simulink model "singlestageSimu"  (R2015b)
settings: Solver=ode45  StartTime=0.0  StopTime=10.0  RelTol=1e-3
values from neighbouring files (symbols this model uses):
  b1n = 0.9    [directComputeTF.m]
  b2n = 0.8    [directComputeTF.m]
libraries: fl_lib x9, nesl_utility x3
settings Model: Creator=Jinwen  LastModifiedBy=Jinwen
settings DataIOCC: SaveFormat=Array
settings HardwareCC: ProdBitPerPointer=32  ProdLargestAtomicFloat=None  ProdIntDivRoundTo=Undefined  ProdEndianess=Unspecified  ProdWordSize=32  ProdHWDeviceType=32-bit Generic
settings GRTTargetCC: GeneratePreprocessorConditionals=Disable all
settings ConfigComp: CovModelRefEnable=Off

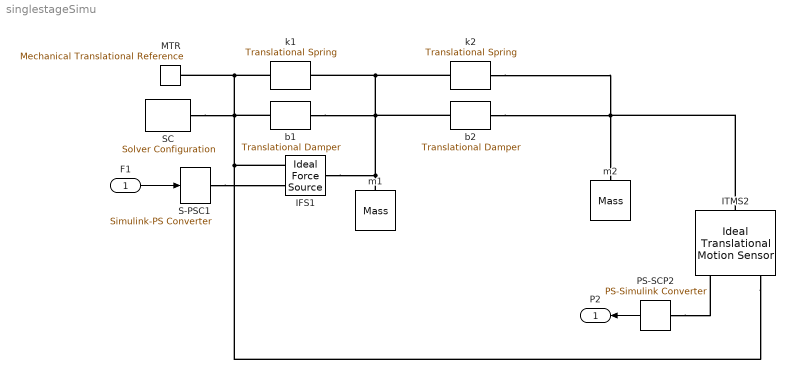
== system singlestageSimu ==
  F1 : Inport
  IFS1 : fl_lib/Mechanical/Mechanical Sources/Ideal Force Source
  ITMS2 : fl_lib/Mechanical/Mechanical Sensors/Ideal Translational Motion Sensor  offset=0 m
  MTR : fl_lib/Mechanical/Translational Elements/Mechanical Translational Reference
  PS-SCP2 : nesl_utility/PS-Simulink Converter  PhysicalDomain=network_engine_domain  SubClassName=ps_output  LeftPortType=input  RightPortType=output  PseudoPeriodic=off  Frequencies=[]  Unit=1  AffineConversion=off
  S-PSC1 : nesl_utility/Simulink-PS Converter  PhysicalDomain=network_engine_domain  SubClassName=ps_input  LeftPortType=input  RightPortType=output  PseudoPeriodic=off  Frequencies=[]  NoiseDistribution=none  NoiseParameters=[]  Unit=1  AffineConversion=off  InputFiltering=off  SimscapeFilterOrder=1  InputFilterTimeConstant=0.001  UdotUserProvided=1
  SC : nesl_utility/Solver Configuration  PhysicalDomain=network_engine_domain  SubClassName=solver  LeftPortType=input  RightPortType=generic  Accelerate=off  Tones=[]  Harmonics=[]  SimulateNoise=off  Profile=off  UseLocalSampling=off  EnableSwitchedLinearOptims=on  FrequencyDomain=off  UseCCode=off  RelTol=0.001  AbsTol=1e-06  MinStep=1e-09  ToWorkspace=off  RevertToSquareIcSolve=off  NumHomotopyIterations=100  PhasorMode=off  PhasorModeNumHarmonics=1  DoDC=off  ResidualTolerance=1e-09  UseLocalSolver=off  LocalSolverChoice=NE_BACKWARD_EULER_ADVANCER  LocalSolverSampleTime=0.001  DoFixedCost=off  MaxNonlinIter=3  MaxModeIter=2  LinearAlgebra=Sparse  DelaysMemoryBudget=1024  AutomaticFiltering=on  FilteringTimeConstant=0.001
  b1 : fl_lib/Mechanical/Translational Elements/Translational Damper  D=b1n N/(m/s)  v_specify=off  v_priority=High  v=0 m/s  f_specify=off  f_priority=High  f=0 N
  b2 : fl_lib/Mechanical/Translational Elements/Translational Damper  D=b2n N/(m/s)  v_specify=off  v_priority=High  v=0 m/s  f_specify=off  f_priority=High  f=0 N
  k1 : fl_lib/Mechanical/Translational Elements/Translational Spring  spr_rate=k1n N/m  v_specify=off  v_priority=High  v=0 m/s  f_specify=off  f_priority=High  f=0 N  x_specify=off  x_priority=High  x=0 m
  k2 : fl_lib/Mechanical/Translational Elements/Translational Spring  spr_rate=k2n N/m  v_specify=off  v_priority=High  v=0 m/s  f_specify=off  f_priority=High  f=0 N  x_specify=off  x_priority=High  x=0 m
  m1 : fl_lib/Mechanical/Translational Elements/Mass  mass=m1n kg  v_specify=on  v_priority=High  v=0 m/s  f_specify=on  f_priority=High  f=0 N
  m2 : fl_lib/Mechanical/Translational Elements/Mass  mass=m2n kg  v_specify=on  v_priority=High  v=0 m/s  f_specify=on  f_priority=High  f=0 N
  P2 : Outport
  wires:
  F1/1 -> S-PSC1/1
  PS-SCP2/1 -> P2/1
  connections:
  b1/LConn1 -- b2/RConn1 -- IFS1/LConn1 -- m1/LConn1 -- k2/RConn1 -- k1/LConn1
  b1/RConn1 -- ITMS2/RConn1 -- IFS1/RConn2 -- SC/RConn1 -- k1/RConn1 -- MTR/LConn1
  S-PSC1/RConn1 -- IFS1/RConn1
  k2/LConn1 -- ITMS2/LConn1 -- b2/LConn1 -- m2/LConn1
  PS-SCP2/LConn1 -- ITMS2/RConn3
